simulink model "counter"  (R2024b)
settings: Solver=FixedStepAuto  StartTime=0.0  StopTime=10.0  FixedStep=1  RelTol=1e-3
settings Model: Creator=z004f2se  LastModifiedBy=z004f2se

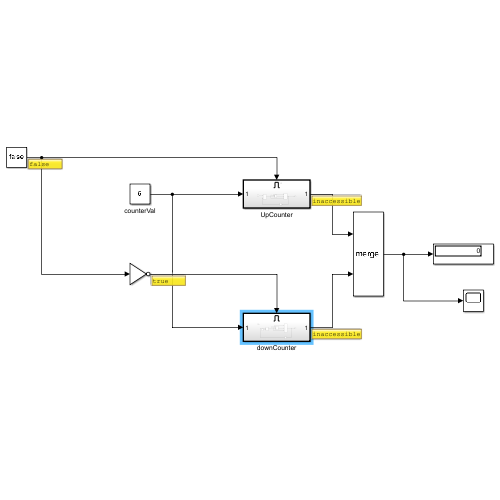
[thumbnail: Simulink's stored preview of the top-level diagram]
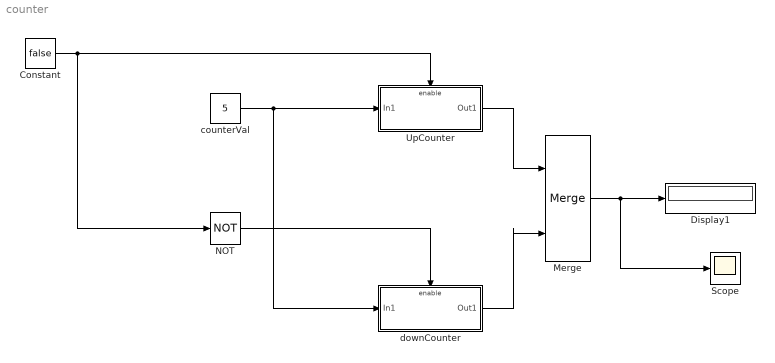
== system counter ==
  Constant : Constant  Value=false
  Display1 : Display
  Merge : Merge
  NOT : Logic  Operator=NOT  IconShape=distinctive  AllPortsSameDT=off  OutDataTypeStr=boolean
  Scope : Scope
  UpCounter : Subsystem  TreatAsAtomicUnit=on
  counterVal : Constant  Value=5
  downCounter : Subsystem  TreatAsAtomicUnit=on
  wires:
  Constant/1 -> NOT/1, UpCounter/Enable
  counterVal/1 -> downCounter/1(In1), UpCounter/1(In1)
  NOT/1 -> downCounter/Enable
  UpCounter/1(Out1) -> Merge/1
  downCounter/1(Out1) -> Merge/2
  Merge/1 -> Scope/1, Display1/1

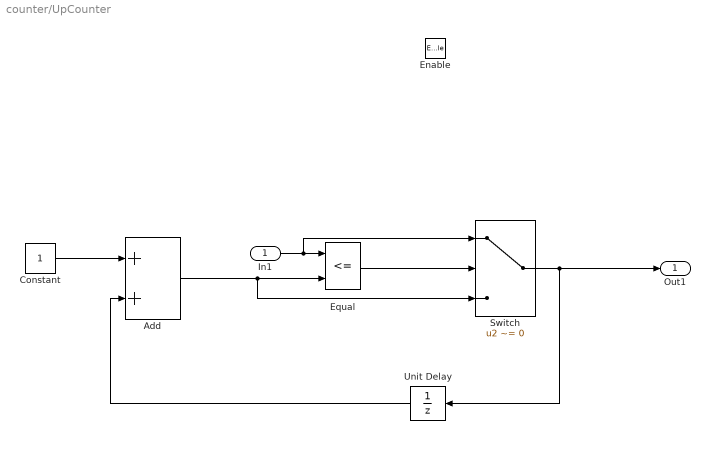
== system counter/UpCounter ==
  In1 : Inport
  Enable : EnablePort
  Add : Sum
  Constant : Constant
  Equal : RelationalOperator  Operator=<=  OutDataTypeStr=boolean  RndMeth=Simplest  InputSameDT=off
  Switch : Switch  Criteria=u2 ~= 0  SaturateOnIntegerOverflow=off  InputSameDT=off
  Unit Delay : UnitDelay  InitialCondition=1  SampleTime=-1  HasFrameUpgradeWarning=on
  Out1 : Outport
  wires:
  Switch/1 -> Out1/1, Unit Delay/1
  Equal/1 -> Switch/2
  Unit Delay/1 -> Add/2
  Constant/1 -> Add/1
  In1/1 -> Switch/1, Equal/1
  Add/1 -> Switch/3, Equal/2

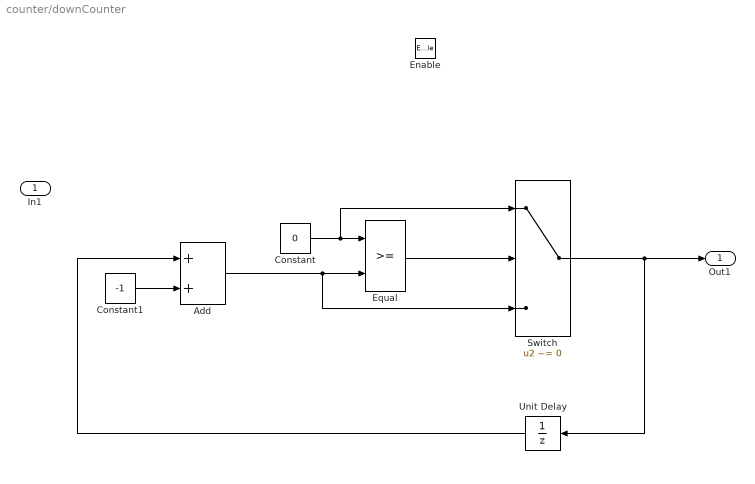
== system counter/downCounter ==
  In1 : Inport
  Enable : EnablePort
  Add : Sum
  Constant : Constant  Value=0
  Constant1 : Constant  Value=-1
  Equal : RelationalOperator  OutDataTypeStr=boolean  RndMeth=Simplest  InputSameDT=off
  Switch : Switch  Criteria=u2 ~= 0  SaturateOnIntegerOverflow=off  InputSameDT=off
  Unit Delay : UnitDelay  InitialCondition=6  SampleTime=-1  HasFrameUpgradeWarning=on
  Out1 : Outport
  wires:
  Equal/1 -> Switch/2
  Constant/1 -> Switch/1, Equal/1
  Add/1 -> Switch/3, Equal/2
  Unit Delay/1 -> Add/1
  Switch/1 -> Out1/1, Unit Delay/1
  Constant1/1 -> Add/2
